simulink model "PositionControl_v2"  (R2023a)
settings: Solver=FixedStepDiscrete  StartTime=0.0  StopTime=inf  FixedStep=0.01  RelTol=1e-3  EnableMultiTasking=on
undefined symbols (not defined in the file or in its folder): DiscIntNeverNeededParam
libraries: M5Core_Library x2, simulink x1
settings Model: ExtModeTrigDuration=2  Creator=auw_a  LastModifiedBy=auw_a
settings OptimizationCC: EnhancedBackFolding=on  PassReuseOutputArgsAs=Individual arguments  ZeroExternalMemoryAtStartup=off  ZeroInternalMemoryAtStartup=off  MaxStackSize=64  OptimizeBlockOrder=speed  DifferentSizesBufferReuse=on  OptimizationCustomize=off  EfficientTunableParamExpr=on
settings DebuggingCC: ParameterOverflowMsg=none  ParameterTunabilityLossMsg=error
settings HardwareCC: ProdBitPerPointer=32  ProdBitPerSizeT=32  ProdBitPerPtrDiffT=32  ProdLargestAtomicInteger=Long  ProdLargestAtomicFloat=Double  ProdWordSize=32  ProdHWDeviceType=ARM Compatible->ARM Cortex
settings SFSimCC: MATLABDynamicMemAlloc=off
settings RTWCC: Description=Embedded Coder  SystemTargetFile=ert.tlc  HardwareBoard=ESP32-WROOM(Arduino Compatible)  TLCOptions="-aInlineSetEventsForThisBaseRateFcn=TLC_FALSE -aSuppressMultiTaskScheduler=TLC_FALSE  -aRateBasedStepFcn=0"  TemplateMakefile=ert_default_tmf  Toolchain=ESP32  BuildConfiguration=Faster Runs
settings CodeAppCC: ForceParamTrailComments=on  IgnoreCustomStorageClasses=off  OperatorAnnotations=on  SimulinkDataObjDesc=on  SFDataObjDesc=on  InsertBlockDesc=on
settings ERTTargetCC: SupportContinuousTime=on  SupportVariableSizeSignals=on  ExtModeTransport=3  ExtModeStaticAlloc=on  ExtModeAutomaticAllocSize=off  ExtModeStaticAllocSize=65536  ExtModeMexFile=ext_xcp  ExtModeIntrfLevel=Level2 - Open

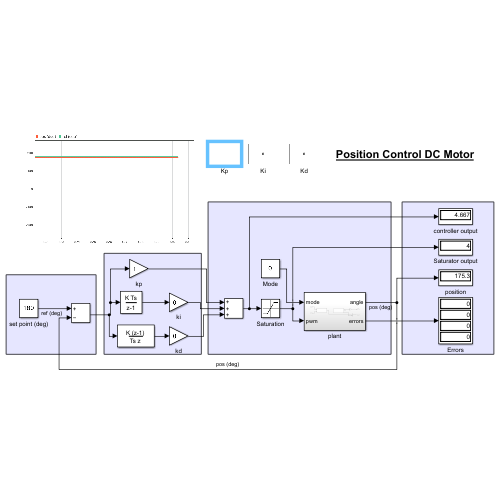
[thumbnail: Simulink's stored preview of the top-level diagram]
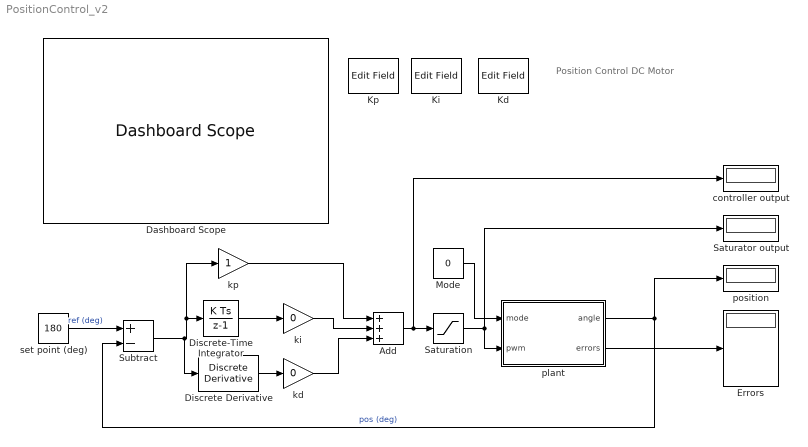
== system PositionControl_v2 ==
  note: Position Control DC Motor
  Add : Sum  Inputs=+++
  Dashboard Scope : DashboardScope  TimeSpan=10  Ymin=-270  Ymax=270  ScaleAtStop=off  UpdateMode=Scroll
  Discrete Derivative : simulink/Discrete/Discrete Derivative  gainval=1.0  ICPrevScaledInput=0.0  OutMin=[]  OutMax=[]  OutDataType=fixdt(1, 16)  OutScaling=2^-10  DoSatur=off
  Discrete-Time Integrator : DiscreteIntegrator  SampleTime=-1  ICPrevOutput=DiscIntNeverNeededParam  ICPrevScaledInput=DiscIntNeverNeededParam
  Errors : Display
  Kd : EditField  LabelPosition=Hide  ShowInitialText=on  Alignment=Center
  Ki : EditField  LabelPosition=Hide  ShowInitialText=on  Alignment=Center
  Kp : EditField  LabelPosition=Hide  ShowInitialText=on  Alignment=Center
  Mode : Constant  Value=0
  Saturation : Saturate  UpperLimit=127  LowerLimit=-127  OutDataTypeStr=int8
  Saturator output : Display
  Subtract : Sum  Inputs=+-
  controller output : Display
  kd : Gain  Gain=0
  ki : Gain  Gain=0
  kp : Gain
  plant : Subsystem
  position : Display
  set point (deg) : Constant  Value=180  OutDataTypeStr=int32  SampleTime=-1
  wires:
  Mode/1 -> plant/1(mode)
  Saturation/1 -> plant/2(pwm), Saturator output/1
  plant/2(errors) -> Errors/1
  Subtract/1 -> Discrete Derivative/1, kp/1, Discrete-Time Integrator/1
  plant/1(angle) -> position/1, Subtract/2  "pos (deg)"
  set point (deg)/1 -> Subtract/1  "ref (deg)"
  Discrete-Time Integrator/1 -> ki/1
  kp/1 -> Add/1
  ki/1 -> Add/2
  Add/1 -> controller output/1, Saturation/1
  kd/1 -> Add/3
  Discrete Derivative/1 -> kd/1

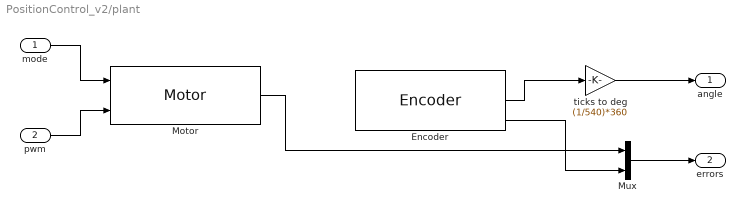
== system PositionControl_v2/plant ==
  mode : Inport
  pwm : Inport  Port=2
  Encoder : M5Core_Library/Encoder  M5_motor=3  s=0.01
  Motor : M5Core_Library/Motor  M5_motor=M3
  Mux : Mux  Inputs=2
  ticks to deg : Gain  Gain=(1/540)*360
  angle : Outport
  errors : Outport  Port=2
  wires:
  Motor/1 -> Mux/1
  Mux/1 -> errors/1
  Encoder/2 -> ticks to deg/1
  ticks to deg/1 -> angle/1
  mode/1 -> Motor/1
  pwm/1 -> Motor/2
  Encoder/3 -> Mux/2
